simulink model "hydrogen_fuel_cell"  (R2023a)
settings: Solver=VariableStepAuto  StartTime=0.0  StopTime=1  RelTol=1e-3
libraries: spsCurrentMeasurementLib x1, spsFuelCellStackLib x1, spsSeriesRLCLoadLib x1, sps_lib x1
settings Model: Creator=vaibhav kumar  LastModifiedBy=vaibhav kumar

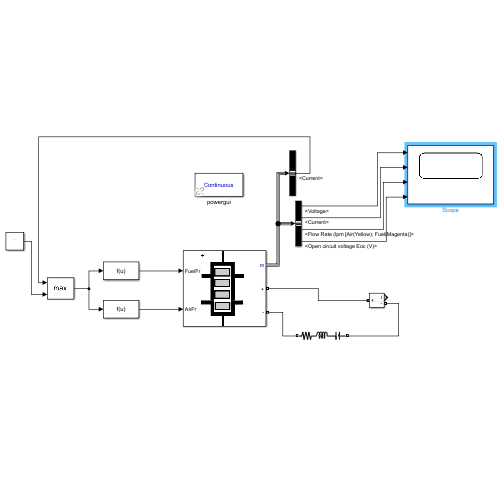
[thumbnail: Simulink's stored preview of the top-level diagram]
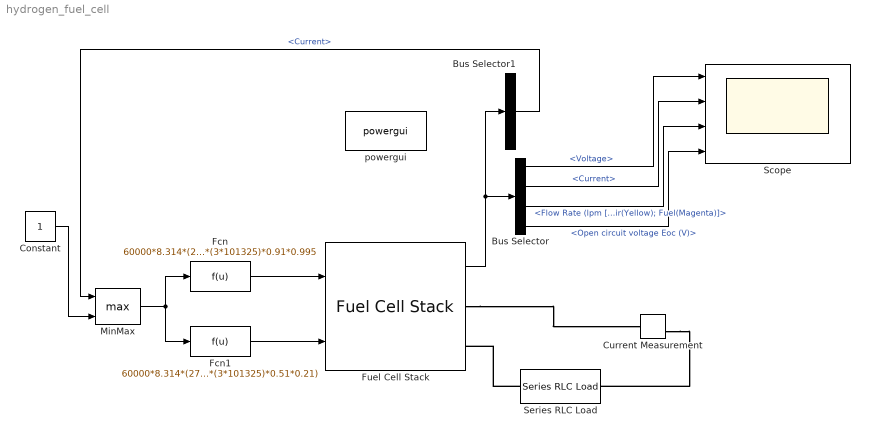
== system hydrogen_fuel_cell ==
  Bus Selector : BusSelector  OutputSignals=Voltage,Current,Flow Rate (lpm [Air(Yellow); Fuel(Magenta)],Open circuit voltage Eoc (V)
  Bus Selector1 : BusSelector  OutputSignals=Current
  Constant : Constant
  Current Measurement : spsCurrentMeasurementLib/Current Measurement  PhasorSimulation=off  OutputType=Complex  PSBequivalent=0
  Fcn : Fcn  Expr=60000*8.314*(273+50)*400*u(1)/2*96500*(3*101325)*0.91*0.995
  Fcn1 : Fcn  Expr=60000*8.314*(273+50)*400*u(1)/(4*96500*(3*101325)*0.51*0.21)
  Fuel Cell Stack : spsFuelCellStackLib/Fuel Cell Stack  PresetModel=No (User-Defined)  FcType=0  Detailed=Detailed  Eoc=[900 895]  NomVI=[80 625]  EndVI=[280 430]  Nc=400  n=80  TOp=50  AirFr=2100  SuppPress=[1.5,1]  Comp=[99.95,21,1]  SignX=off  SignY=off  FlowRateH2=on  FlowRateAir=on  SystemTemp=off  SystemPH2=off  SystemPAir=off  FCDyn=off  FC_tau=1  Peak_O2=80  V_Under=10
      settings: LibrarySourceBlock=sps_lib/Sources/Fuel Cell Stack
  MinMax : MinMax  Function=max  Inputs=2
  Scope : Scope  NumInputPorts=4
  Series RLC Load : spsSeriesRLCLoadLib/Series RLC Load  LConnTagsString=a  RConnTagsString=__new0  NominalVoltage=1000  NominalFrequency=60  ActivePower=10e3  InductivePower=100  CapacitivePower=100  Setx0=off  InitialVoltage=0  SetiL0=off  InitialCurrent=0  Measurements=None  LoadType=constant Z
  powergui : sps_lib/powergui  Priority=1  SimulationMode=Continuous  SampleTime=50e-6  frequency=60  Iterations=50  frequencyindice=0  Pbase=100e6  ErrMax=1e-4  UnitsV=kV  UnitsW=MW  buscounter=0  FunctionMessages=off  echomessages=off  EnableUseOfTLC=off  CurrentSourceSwitches=off  DisableSnubberDevices=off  DisableRonSwitches=off  DisableVfSwitches=off  DisplayEquations=off  AutomaticDiscreteSolvers=off  SolverType=Tustin/Backward Euler (TBE)  Interpol=off  ExternalGateDelay=off  methode=off  Ts=100  x0status=blocks  SPID=on  SwTol=0  HookPort=off  NonlinearTolerance=1e-4  nMaxIteration=100  ContinueOnMaxIteration=off  RestoreLinks=warning  ResistiveCurrentMeasurement=off  Frange=[0:2:500]  Ylog=off  Xlog=on  ShowGrid=off  save=off  variable=ZData  structure=0  ZoomFFT=off  StartTime=0.0  cycles=1  DisplayStyle=1  fundamental=60  FreqAxis=off  MaxFrequency=1000  frequencyindicesteady=1  RmsSteady=1  display=off
  wires:
  Fcn/1 -> Fuel Cell Stack/1
  Fcn1/1 -> Fuel Cell Stack/2
  Fuel Cell Stack/1 -> Bus Selector1/1, Bus Selector/1
  Bus Selector/1 -> Scope/1  "<Voltage>"
  Bus Selector/2 -> Scope/2  "<Current>"
  Bus Selector/3 -> Scope/3  "<Flow Rate (lpm [Air(Yellow); Fuel(Magenta)]>"
  Bus Selector/4 -> Scope/4  "<Open circuit voltage Eoc (V)>"
  Bus Selector1/1 -> MinMax/1  "<Current>"
  Constant/1 -> MinMax/2
  MinMax/1 -> Fcn1/1, Fcn/1
  connections:
  Fuel Cell Stack/RConn1 -- Current Measurement/LConn1
  Current Measurement/RConn1 -- Series RLC Load/RConn1
  Series RLC Load/LConn1 -- Fuel Cell Stack/RConn2
